simulink model "main"  (R2020a)
settings: Solver=ode2  StartTime=0.0  StopTime=24  FixedStep=T_simulation  RelTol=1e-3
model workspace (MAT data in the model file):
  B_bobine = 0.1128
  K_L = 0.004
  K_bobine = 0.8493
  K_c = 1.422
  K_e = 0.9495
  K_pos = 806.5
  Ki = 0.1408
  Kp = 0.001
  N_bobine = 66
  T_simulation = 9.09090909091e-05
  V_consigne = 1.8
  a = 0.000197
  adc_entrees_resolution = 10
  b = 0.0001263
  dac_commande_resolution = 12
  f_courant = 7.8
  f_echant = 22
  f_position = 7.8
  g = 9.81
  m_etalon_max = 100
  m_etalon_min = 0
  m_lame = 150
  r_bobine = 0.0203
  tau_L = 0.1
  v_pos_max = 4.88
  v_pos_min = 0.608
  x_max = 0.0031
  x_min = -0.0031
libraries: simulink x2
settings Model: OrderedModelArguments=off  Creator=freud  LastModifiedBy=frfoc1

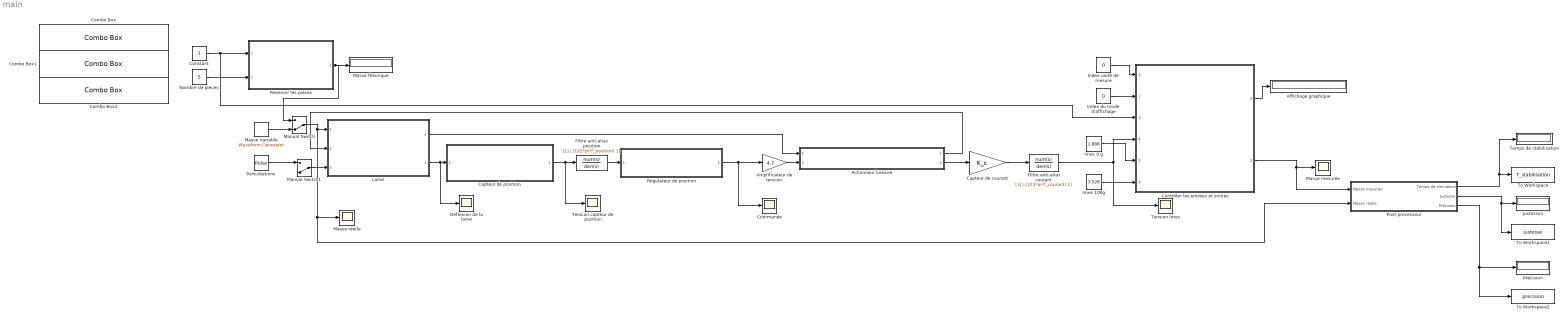
== system main ==
  Actionneur linéaire : Subsystem  ReferencedSubsystem=Actionneur_lineaire  L_bobine=212  R_bobine=1.424  R_eq=1.1
  Affichage graphique : Display
  Amplificateur de tension : Gain  Gain=4.7
  Capteur de courant : Gain  Gain=K_c
  Capteur de position : Subsystem  ReferencedSubsystem=Mesurer_la_position_de_la_lame
  Combo Box : ComboBox  SelectedLabel=10 ¢
      settings: Values={{'5 ¢', '10 ¢', '25 ¢', '1 $', '2 $'}, [0 1 2 3 4]}
  Combo Box1 : ComboBox  SelectedLabel=Grammes
      settings: Values={{'Grammes', 'Onces'}, [0 1]}
  Combo Box2 : ComboBox  SelectedLabel=Afficher la masse
      settings: Values={{'Compter les pièces', 'Afficher la masse'}, [1 0]}
  Commande : Scope
  Constant : Constant
  Contrôler les entrées et sorties : Subsystem  ReferencedSubsystem=Controler_les_entrees_et_sorties  NombreDePiecesMax=10  B=0.1128  r=0.0203  N=66  K_c=1.422
  Déflexion de la lame : Scope
  Filtre anti-alias courant : TransferFcn  Denominator=[1/(2*pi*f_courant) 1]  mask{f_courant=f_echant/2}
      mask prompts: f_courant "Fréquence de coupure (Hz)"
  Filtre anti-alias position : TransferFcn  Denominator=[1/(2*pi*f_position) 1]  mask{f_position=f_echant/4}
      mask prompts: f_position "Fréquence de coupure (Hz)"
  Imes 0 g : Constant  Value=1.888
  Imes 100g : Constant  Value=3.526
  Index du mode d'affichage : Constant  Value=0
  Index unité de mesure : Constant  Value=0
  Justesse1 : Display
  Lame : Subsystem  ReferencedSubsystem=Lame
      settings: PortSchema="{\"entries\":[{\"content\":{\"sides\":[{\"content\":{\"connectorIds\":[\"In1\",\"In2\",\"In3\"]},\"type\":\"ConnectorPlacement.EquallySpacedRectSide\",\"uuid\":\"2a4045bc-55b2-4393-8a6c-c314e497dd61\"},{\"content\":{\"connectorIds\":[\"Out2\",\"Out1\"],\"side\":\"RIGHT\"},\"type\":\"ConnectorPlacement.EquallySpacedRectSide\",\"uuid\":\"257aae75-8186-40ca-b52a-acd04e564c85\"},{\"content\":{\"connectorIds\":[],\"side\":\"TOP\"},\"type\":\"ConnectorPlacement.EquallySpacedRectSide\",\"uuid\":\"414cd986-f566-40b5-926a-0680dd19a9a1\"}]},\"type\":\"ConnectorPlacement.EquallySpacedConnector\",\"uuid\":\"94073dfc-1906-44b0-91f9-39d1a5aeb319\"}],\"packageUris\":[\"http://schema.mathworks.com/mf0/Connector/19700101\"],\"version\":\"1.0\"}"
  Manual Switch : ManualSwitch  CurrentSetting=0
  Manual Switch1 : ManualSwitch  CurrentSetting=0
  Masse Variable : simulink/Sources/Waveform Generator  OutMin=[]  OutMax=[]  OutDataTypeStr=double  SelectedSignal=3  Signals=step('StepTime',10,'InitialValue',85,'FinalValue',35)#50#step('StepTime',10,'InitialValue',0,'FinalValue',100)+step('StepTime',20,'InitialValue',0,'FinalValue',-100)  BlockNames=MultiportSwitch_46f68ba5669b4dc#MultiportSwitch_59ed0b4f51684cb#MultiportSwitch_c08e21cbed45463  SampleTime=0.1
  Masse mesurée : Scope
  Masse réelle : Scope
  Masse théorique : Display
  Nombre de pièces : Constant  Value=5
  Perturbations : DiscretePulseGenerator  PulseType=Time based  Amplitude=0  Period=15  PulseWidth=9
  Post-processeur : Subsystem
  Précision : Display
  Recevoir les pièces : Subsystem  ReferencedSubsystem=Recevoir_les_pieces
  Régulateur de position : Subsystem  ReferencedSubsystem=Regulateur_de_position
  Temps de stabilisation : Display
  Tension Imes : Scope
  Tension capteur de position : Scope
  To Workspace : ToWorkspace  VariableName=T_stabilisation  SampleTime=-1
      settings: MaxDataPoints=1
  To Workspace1 : ToWorkspace  VariableName=justesse  SampleTime=-1
      settings: MaxDataPoints=1
  To Workspace2 : ToWorkspace  VariableName=precision  SampleTime=-1
      settings: MaxDataPoints=1
  wires:
  Actionneur linéaire/1 -> Lame/2
  Recevoir les pièces/1 -> Manual Switch/1, Masse théorique/1
  Index du mode d'affichage/1 -> Contrôler les entrées et sorties/2
  Index unité de mesure/1 -> Contrôler les entrées et sorties/1
  Contrôler les entrées et sorties/1 -> Affichage graphique/1
  Lame/1 -> Déflexion de la lame/1, Capteur de position/1
  Lame/2 -> Actionneur linéaire/1
  Capteur de courant/1 -> Filtre anti-alias courant/1
  Filtre anti-alias courant/1 -> Tension Imes/1, Contrôler les entrées et sorties/4
  Capteur de position/1 -> Tension capteur de position/1, Filtre anti-alias position/1
  Nombre de pièces/1 -> Recevoir les pièces/2
  Constant/1 -> Contrôler les entrées et sorties/3, Recevoir les pièces/1
  Masse Variable/1 -> Manual Switch/2
  Manual Switch/1 -> Lame/1, Masse réelle/1, Post-processeur/2(Masse réelle)
  Manual Switch1/1 -> Lame/3
  Perturbations/1 -> Manual Switch1/1
  Contrôler les entrées et sorties/2 -> Masse mesurée/1, Post-processeur/1(Masse mesurée)
  Post-processeur/2(Justesse) -> To Workspace1/1, Justesse1/1
  Post-processeur/1(Temps de simulation) -> Temps de stabilisation/1, To Workspace/1
  Post-processeur/3(Précision) -> To Workspace2/1, Précision/1
  Amplificateur de tension/1 -> Actionneur linéaire/2
  Actionneur linéaire/2 -> Capteur de courant/1
  Filtre anti-alias position/1 -> Régulateur de position/1
  Régulateur de position/1 -> Commande/1, Amplificateur de tension/1
  Imes 0 g/1 -> Contrôler les entrées et sorties/5
  Imes 100g/1 -> Contrôler les entrées et sorties/6

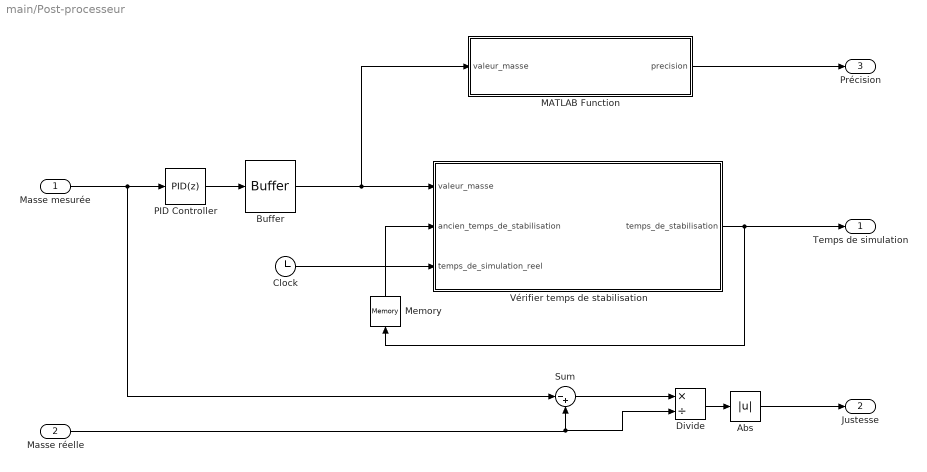
== system main/Post-processeur ==
  Masse mesurée : Inport
  Masse réelle : Inport  Port=2
  Abs : Abs
  Buffer : Buffer  N=f_echant*3  OutputFrames=off
  Clock : Clock
  Divide : Product  Inputs=*/
  MATLAB Function : MATLAB Function  TreatAsAtomicUnit=on
  Memory : Memory
  PID Controller : simulink/Continuous/PID Controller  Controller=PID  Form=Parallel  TimeDomain=Discrete-time  UseExternalTs=off  SampleTime=1/(f_echant*5)  IntegratorMethod=Forward Euler  FilterMethod=Forward Euler  ControllerParametersSource=internal  P=1  I=0  D=0  UseFilter=on  N=100  TunerSelectOption=Transfer Function Based (PID Tuner App)  InitialConditionSource=internal  InitialConditionForIntegrator=0  InitialConditionForFilter=0  DifferentiatorICPrevScaledInput=0  ExternalReset=none  TrackingMode=off  Kt=1  LimitOutput=off  UpperSaturationLimit=inf  LowerSaturationLimit=-inf  LinearizeAsGain=on  AntiWindupMode=none  Kb=1  POutMin=[]  POutMax=[]  IOutMin=[]  IOutMax=[]  DOutMin=[]  DOutMax=[]  NOutMin=[]  NOutMax=[]  SumOutMin=[]  SumOutMax=[]  SaturationOutMin=[]  SaturationOutMax=[]  PParamMin=[]  PParamMax=[]  IParamMin=[]  IParamMax=[]  DParamMin=[]  DParamMax=[]  NParamMin=[]  NParamMax=[]  KbParamMin=[]  KbParamMax=[]  KtParamMin=[]  KtParamMax=[]  KbOutMin=[]  KbOutMax=[]  KtOutMin=[]  KtOutMax=[]  IntegratorOutMin=[]  IntegratorOutMax=[]  FilterOutMin=[]  FilterOutMax=[]  SumI1OutMin=[]  SumI1OutMax=[]  SumI2OutMin=[]  SumI2OutMax=[]  SumI3OutMin=[]  SumI3OutMax=[]  SumI4OutMin=[]  SumI4OutMax=[]  SumDOutMin=[]  SumDOutMax=[]  DifferentiatorOutMin=[]  DifferentiatorOutMax=[]  FilterDiffOutCoefMin=[]  FilterDiffOutCoefMax=[]  ReciprocalOutMin=[]  ReciprocalOutMax=[]  SumDenOutMin=[]  SumDenOutMax=[]  SumNumOutMin=[]  SumNumOutMax=[]  DivideOutMin=[]  DivideOutMax=[]  UdiffTsProdOutMin=[]  UdiffTsProdOutMax=[]  NTsProdOutMin=[]  NTsProdOutMax=[]  UintegralTsProdOutMin=[]  UintegralTsProdOutMax=[]  UngainTsProdOutMin=[]  UngainTsProdOutMax=[]  IntegratorContinuousStateAttributes=''  IntegratorStateMustResolveToSignalObject=off  IntegratorRTWStateStorageClass=Auto  FilterContinuousStateAttributes=''  FilterStateMustResolveToSignalObject=off  FilterRTWStateStorageClass=Auto  ParallelPVariant=InternalParameters  IdealPVariant=Disabled  IVariant=InternalParameters  DVariant=InternalParameters  IntegratorVariant=Discrete  SatVariant=Disabled  AWVariant=Passthrough  PCopyVariant=Disabled  TRVariant=Disabled  FdbkBlocksVariant=Forward  IdealPFdbkVariant=Disabled  SatFdbkVariant=Disabled  DerivativeFilterVariant=ForwardEulerFilter  NVariant=InternalParameters  NCopyVariant=Disabled  FilterICVariant=InternalICsFilter  IntegratorICVariant=InternalICs  ExternalResetVariant=Disabled  TRSumVariant=Passthrough  SumFdbkVariant=Disabled  SumVariant=Sum_PID  TsampFilterVariant=InternalTs  TsampNgainVariant=Passthrough  TsampIntegralVariant=Passthrough
  Sum : Sum  Inputs=|-+
  Vérifier temps de stabilisation : MATLAB Function  TreatAsAtomicUnit=on
  Temps de simulation : Outport
  Justesse : Outport  Port=2
  Précision : Outport  Port=3
  wires:
  Masse mesurée/1 -> Sum/1, PID Controller/1
  Divide/1 -> Abs/1
  Sum/1 -> Divide/1
  Masse réelle/1 -> Divide/2, Sum/2
  Abs/1 -> Justesse/1
  PID Controller/1 -> Buffer/1
  Memory/1 -> Vérifier temps de stabilisation/2(ancien_temps_de_stabilisation)
  Clock/1 -> Vérifier temps de stabilisation/3(temps_de_simulation_reel)
  Buffer/1 -> MATLAB Function/1(valeur_masse), Vérifier temps de stabilisation/1(valeur_masse)
  Vérifier temps de stabilisation/1(temps_de_stabilisation) -> Temps de simulation/1, Memory/1
  MATLAB Function/1(precision) -> Précision/1

== matlab function main/Post-processeur/MATLAB Function ==
  data: valeur_masse input; precision output
function precision = precision(valeur_masse)
    precision = abs(max(valeur_masse(:)) - min(valeur_masse(:)));
end

== matlab function main/Post-processeur/Vérifier temps de stabilisation ==
  data: valeur_masse input; temps_de_stabilisation output; ancien_temps_de_stabilisation input; temps_de_simulation_reel input
function temps_de_stabilisation = get_temps_stabilisation(valeur_masse,ancien_temps_de_stabilisation,temps_de_simulation_reel)
    margeDeStabilite = 0.015;
    Max = max(valeur_masse(:));
    Min = min(valeur_masse(:));
    if margeDeStabilite <= (Max - Min)/Max
        temps_de_stabilisation = temps_de_simulation_reel;
    else
        temps_de_stabilisation = ancien_temps_de_stabilisation;
    end
end
